simulink model "LQR"  (R2023b)
settings: Solver=VariableStepAuto  StartTime=0.0  StopTime=10.0  RelTol=1e-3
values from neighbouring files (symbols this model uses):
  A = sys_pade.A    [attempt.m]    (also in model_approximation.m; observer.m = [-7.9641 0 8.7857; 1.0000 0 0; 0 0 -35.1427]; progetto.m = [0 1; 0 -1/Tm]; tuning.m)
  B = sys_pade.B    [attempt.m]    (also in model_approximation.m; observer.m = [-1;0;8]; progetto.m = [0 ;km/Tm]; tuning.m)
  kr = -1/(C*inv(A-B*K_tilde(1:3))*B)    [controller_tuning.m]    (also in progetto.m = -1/(C*inv(A-B*K)*B); tuning.m)
  r = 50    [progetto.m]
undefined symbols (not defined in the file or in its folder): disturbance, K_tilde
settings Model: Creator=giova  LastModifiedBy=david

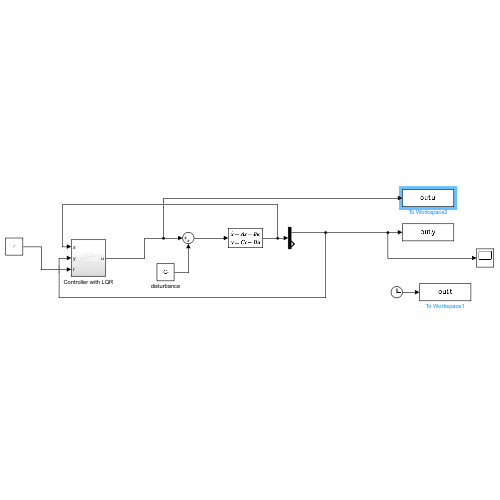
[thumbnail: Simulink's stored preview of the top-level diagram]
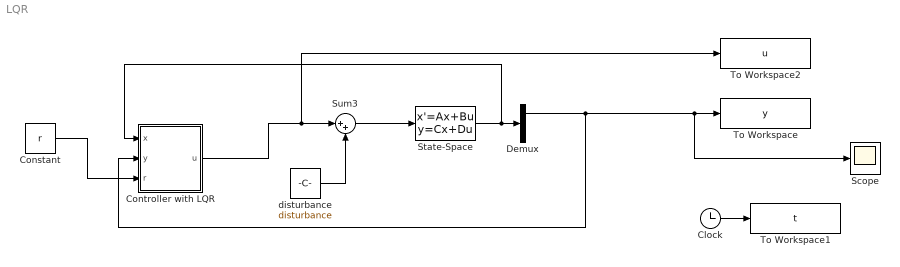
== system LQR ==
  Clock : Clock
  Constant : Constant  Value=r
  Controller with LQR : Subsystem
  Demux : Demux  Outputs=2
  Scope : Scope
  State-Space : StateSpace  A=A  B=B  C=eye(2)  D=[0; 0]  InitialCondition=0
  Sum3 : Sum  Inputs=|++
  To Workspace : ToWorkspace  VariableName=y  SampleTime=-1
  To Workspace1 : ToWorkspace  VariableName=t  SampleTime=-1
  To Workspace2 : ToWorkspace  VariableName=u  SampleTime=-1
  disturbance : Constant  Value=disturbance
  wires:
  State-Space/1 -> Controller with LQR/1(x), Demux/1
  Clock/1 -> To Workspace1/1
  Demux/1 -> Controller with LQR/2(y), Scope/1, To Workspace/1
  Sum3/1 -> State-Space/1
  Constant/1 -> Controller with LQR/3(r)
  Controller with LQR/1(u) -> To Workspace2/1, Sum3/1
  disturbance/1 -> Sum3/2

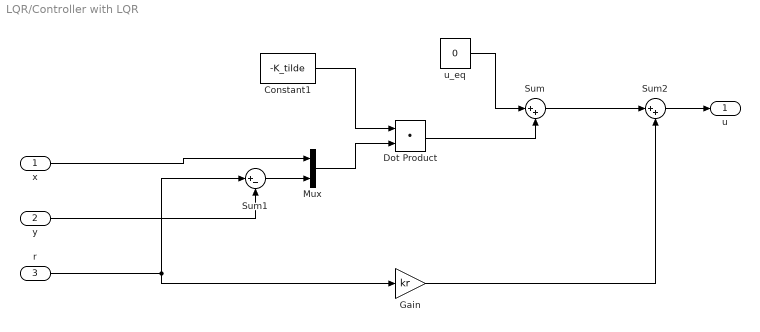
== system LQR/Controller with LQR ==
  x : Inport
  y : Inport  Port=2
  r : Inport  Port=3
  Constant1 : Constant  Value=-K_tilde
  Dot Product : DotProduct  OutDataTypeStr=Inherit: Inherit via internal rule
  Gain : Gain  Gain=kr
  Mux : Mux  Inputs=2
  Sum : Sum  Inputs=|++
  Sum1 : Sum  Inputs=|+-
  Sum2 : Sum  Inputs=|++
  u_eq : Constant  Value=0
  u : Outport
  wires:
  Sum1/1 -> Mux/2
  r/1 -> Sum1/1, Gain/1
  Dot Product/1 -> Sum/2
  Sum/1 -> Sum2/1
  Mux/1 -> Dot Product/2
  u_eq/1 -> Sum/1
  Gain/1 -> Sum2/2
  Constant1/1 -> Dot Product/1
  Sum2/1 -> u/1
  x/1 -> Mux/1
  y/1 -> Sum1/2
